simulink model "QiehuanZongheLianxi"  (Simulink 9.1)
settings: Solver=VariableStepAuto  StartTime=0.0  StopTime=5  RelTol=1e-3
PreLoadFcn:
  | clear
settings Model: Creator=McQueen_Zero  LastModifiedBy=McQueen_Zero
settings DataIOCC: SaveFormat=Dataset
settings OptimizationCC: LifeSpan=auto
settings DebuggingCC: UnderspecifiedInitializationDetection=Simplified  MergeDetectMultiDrivingBlocksExec=error  SFUnexpectedBacktrackingDiag=error  SFNoUnconditionalDefaultTransitionDiag=error  SFExecutionAtInitializationDiag=warning
settings HardwareCC: ProdBitPerPointer=64  ProdBitPerSizeT=64  ProdBitPerPtrDiffT=64  ProdLargestAtomicFloat=Float  ProdIntDivRoundTo=Zero  ProdEndianess=LittleEndian  ProdWordSize=64  ProdHWDeviceType=Intel->x86-64 (Windows64)
settings ModelReferenceCC: PropagateSignalLabelsOutOfModel=on
settings CodeAppCC: StateflowObjectComments=off
settings GRTTargetCC: TargetLangStandard=C99 (ISO)  CombineOutputUpdateFcns=on  GRTInterface=off
settings ConfigComp: CovMetricSettings=dwe  CovHtmlReporting=off  CovSaveCumulativeToWorkspaceVar=off  CovSaveSingleToWorkspaceVar=off  CovExternalEMLEnable=on

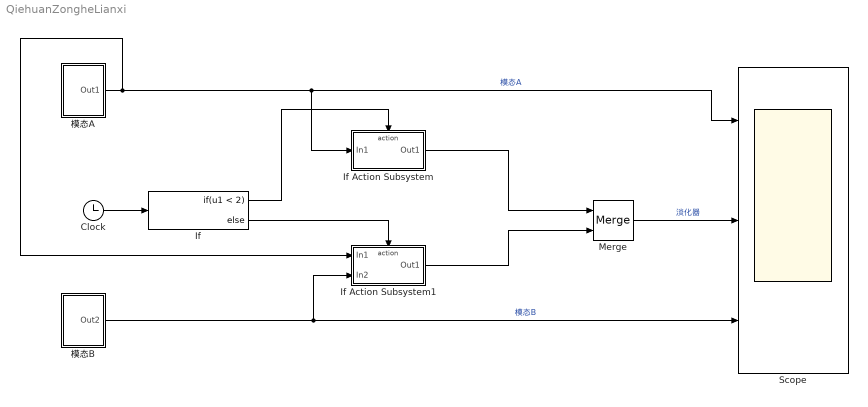
== system QiehuanZongheLianxi ==
  Clock : Clock
  If : If  IfExpression=u1 < 2
  If Action Subsystem : Subsystem  TreatAsAtomicUnit=on
  If Action Subsystem1 : Subsystem  TreatAsAtomicUnit=on
  Merge : Merge
  Scope : Scope  NumInputPorts=3
  模态A : Subsystem  mask{A=1}
      mask prompts: A "模态A的输出"
  模态B : Subsystem  mask{B=2}
      mask prompts: B "模态B的输出"
  wires:
  模态B/1(Out2) -> If Action Subsystem1/2(In2), Scope/3  "模态B"
  模态A/1(Out1) -> Scope/1, If Action Subsystem/1(In1), If Action Subsystem1/1(In1)  "模态A"
  Clock/1 -> If/1
  If/1 -> If Action Subsystem/Action
  If/2 -> If Action Subsystem1/Action
  Merge/1 -> Scope/2  "淡化器"
  If Action Subsystem1/1(Out1) -> Merge/2
  If Action Subsystem/1(Out1) -> Merge/1

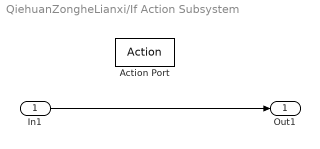
== system QiehuanZongheLianxi/If Action Subsystem ==
  In1 : Inport
  Action Port : ActionPort  ActionType=then
  Out1 : Outport
  wires:
  In1/1 -> Out1/1

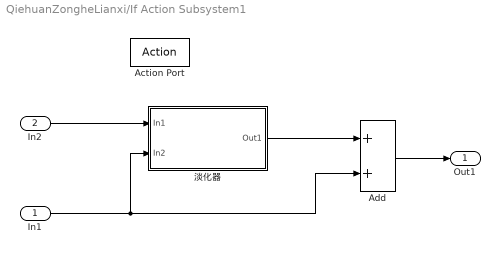
== system QiehuanZongheLianxi/If Action Subsystem1 ==
  In1 : Inport
  In2 : Inport  Port=2
  Action Port : ActionPort  ActionType=else
  Add : Sum
  淡化器 : Subsystem  mask{ts=2}
      mask prompts: ts "淡化器时间ts"
  Out1 : Outport
  wires:
  In1/1 -> Add/2, 淡化器/2(In2)
  Add/1 -> Out1/1
  In2/1 -> 淡化器/1(In1)
  淡化器/1(Out1) -> Add/1

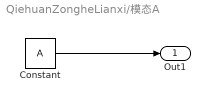
== system QiehuanZongheLianxi/模态A ==
  Constant : Constant  Value=A
  Out1 : Outport
  wires:
  Constant/1 -> Out1/1

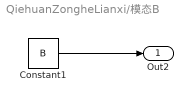
== system QiehuanZongheLianxi/模态B ==
  Constant1 : Constant  Value=B
  Out2 : Outport
  wires:
  Constant1/1 -> Out2/1

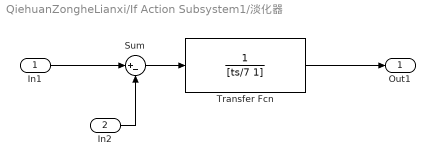
== system QiehuanZongheLianxi/If Action Subsystem1/淡化器 ==
  In1 : Inport
  In2 : Inport  Port=2
  Sum : Sum  Inputs=|+-
  Transfer Fcn : TransferFcn  Denominator=[ts/7 1]
  Out1 : Outport
  wires:
  In1/1 -> Sum/1
  Sum/1 -> Transfer Fcn/1
  In2/1 -> Sum/2
  Transfer Fcn/1 -> Out1/1
